simulink model "mbed_nucleo_f767_RTOS_blinky"  (R2015a)
settings: Solver=FixedStepDiscrete  SolverMode=SingleTasking  StartTime=0.0  StopTime=10.0  FixedStep=1e-3  RelTol=1e-3
libraries: mbed_lib x3, simulink x1
settings Model: Creator=oh  LastModifiedBy=oh
settings OptimizationCC: OptimizeModelRefInitCode=on  LifeSpan=1
settings HardwareCC: ProdLargestAtomicInteger=Long  ProdLargestAtomicFloat=Double  ProdEndianess=LittleEndian  ProdHWDeviceType=ARM Compatible->ARM Cortex
settings RTWCC: SystemTargetFile=mbed.tlc  TemplateMakefile=mbed.tmf  Description=Mbed Target (Embedded Target)  TargetLang=C++
settings CodeAppCC: IgnoreCustomStorageClasses=off
settings STFCustomTargetCC: CombineOutputUpdateFcns=on  SupportContinuousTime=off  SupportVariableSizeSignals=off  SystemTargetFile=mbed.tlc
settings ERTTargetCC: SupportContinuousTime=off  SupportVariableSizeSignals=off  ERTCustomFileTemplate=mbed_file_process.tlc

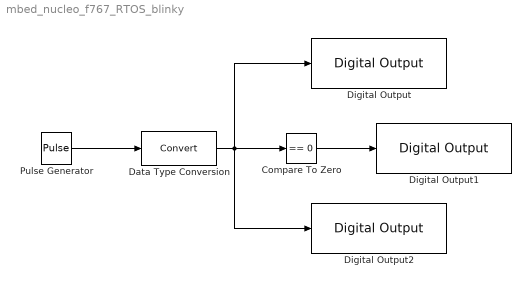
== system mbed_nucleo_f767_RTOS_blinky ==
  Compare To Zero : simulink/Logic and Bit Operations/Compare To Zero  relop===  OutDataTypeStr=uint8
  Data Type Conversion : DataTypeConversion
  Digital Output : mbed_lib/GPIO/Digital Output  SParameter2=B  SParameter1=0  SParameter3=PullDefault  SampleTime=-1
  Digital Output1 : mbed_lib/GPIO/Digital Output  SParameter2=B  SParameter1=7  SParameter3=PullDefault  SampleTime=-1
  Digital Output2 : mbed_lib/GPIO/Digital Output  SParameter2=B  SParameter1=14  SParameter3=PullDefault  SampleTime=-1
  Pulse Generator : DiscretePulseGenerator  PulseType=Time based  Period=0.5  PulseWidth=50
  wires:
  Pulse Generator/1 -> Data Type Conversion/1
  Data Type Conversion/1 -> Digital Output/1, Digital Output2/1, Compare To Zero/1
  Compare To Zero/1 -> Digital Output1/1
